simulink model "template_KR4_PreRTHS"  (Simulink 8.2)
settings: Solver=FixedStepDiscrete  StartTime=0.0  StopTime=RunningTime  FixedStep=sample  RelTol=1e-3
undefined symbols (not defined in the file): ElementsStruct, Integrator, NumFreeDOF, RigidLinkMasterMatrix, RigidLinkNo, RigidLinkNodeID, RigidLinkSlaveMatrix, sample, SampleRate, Structure
libraries: HybridFEMLibrary x2
(part 1 of 2)
CloseFcn:
  | rtwprivate ssgencode ModelCloseRequest hybriddaq1dof
settings Model: MinMaxOverflowLogging=ForceOff  Creator=RTMD  LastModifiedBy=Thomas Marullo  BufferReuse=off
settings DataIOCC: LimitDataPoints=off
settings OptimizationCC: BlockReduction=off  OptimizeBlockIOStorage=off  BufferReuse=off  ExpressionFolding=off  LocalBlockOutputs=off  InitFltsAndDblsToZero=on
settings DebuggingCC: SignalResolutionControl=TryResolveAllWithWarning  MultiTaskDSMMsg=warning  FcnCallInpInsideContextMsg=EnableAllAsWarning
settings HardwareCC: ProdIntDivRoundTo=Zero  ProdEndianess=LittleEndian  ProdHWDeviceType=Generic->32-bit x86 compatible
settings SFSimCC: SimParseCustomCode=off
settings RTWCC: ProcessScript=grt_make_rtw_hook
settings GRTTargetCC: CombineOutputUpdateFcns=on  GRTInterface=off

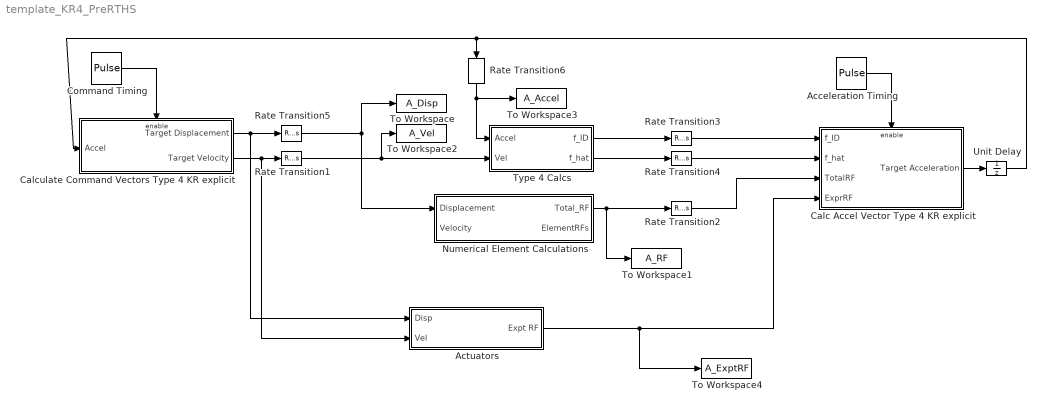
== system template_KR4_PreRTHS ==
  Acceleration Timing : DiscretePulseGenerator  Period=Integrator.Interpolations  PhaseDelay=Integrator.Interpolations-1  SampleTime=sample
  Actuators : Subsystem
  Calc Accel Vector Type 4 KR explicit : Subsystem
  Calculate Command Vectors Type 4 KR explicit : Subsystem  TreatAsAtomicUnit=on  SystemSampleTime=SampleRate
  Command Timing : DiscretePulseGenerator  Period=Integrator.Interpolations  SampleTime=sample
  Numerical Element Calculations : MATLAB Function  TreatAsAtomicUnit=on
  Rate Transition1 : RateTransition  Deterministic=off  OutPortSampleTime=SampleRate
  Rate Transition2 : RateTransition  Deterministic=off  OutPortSampleTime=sample
  Rate Transition3 : RateTransition  Deterministic=off  OutPortSampleTime=sample
  Rate Transition4 : RateTransition  Deterministic=off  OutPortSampleTime=sample
  Rate Transition5 : RateTransition  Deterministic=off  OutPortSampleTime=SampleRate
  Rate Transition6 : RateTransition  Deterministic=off  OutPortSampleTime=SampleRate
  To Workspace : ToWorkspace  VariableName=A_Disp  SampleTime=-1
  To Workspace1 : ToWorkspace  VariableName=A_RF  SampleTime=-1
  To Workspace2 : ToWorkspace  VariableName=A_Vel  SampleTime=-1
  To Workspace3 : ToWorkspace  VariableName=A_Accel  SampleTime=-1
  To Workspace4 : ToWorkspace  VariableName=A_ExptRF  SampleTime=-1
  Type 4 Calcs : Subsystem  TreatAsAtomicUnit=on  SystemSampleTime=SampleRate
  Unit Delay : UnitDelay  InitialCondition=Integrator.Acceleration  SampleTime=-1
  wires:
  Acceleration Timing/1 -> Calc Accel Vector Type 4 KR explicit/Enable
  Calculate Command Vectors Type 4 KR explicit/2(Target Velocity) -> Rate Transition1/1, Actuators/2(Vel)
  Rate Transition2/1 -> Calc Accel Vector Type 4 KR explicit/3(TotalRF)
  Command Timing/1 -> Calculate Command Vectors Type 4 KR explicit/Enable
  Calculate Command Vectors Type 4 KR explicit/1(Target Displacement) -> Rate Transition5/1, Actuators/1(Disp)
  Rate Transition5/1 -> Numerical Element Calculations/1(Displacement), To Workspace/1
  Unit Delay/1 -> Rate Transition6/1, Calculate Command Vectors Type 4 KR explicit/1(Accel)
  Rate Transition3/1 -> Calc Accel Vector Type 4 KR explicit/1(f_ID)
  Numerical Element Calculations/1(Total_RF) -> Rate Transition2/1, To Workspace1/1
  Rate Transition1/1 -> Type 4 Calcs/2(Vel), To Workspace2/1
  Calc Accel Vector Type 4 KR explicit/1(Target Acceleration) -> Unit Delay/1
  Type 4 Calcs/1(f_ID) -> Rate Transition3/1
  Type 4 Calcs/2(f_hat) -> Rate Transition4/1
  Rate Transition6/1 -> Type 4 Calcs/1(Accel), To Workspace3/1
  Rate Transition4/1 -> Calc Accel Vector Type 4 KR explicit/2(f_hat)
  Actuators/1(Expt RF) -> To Workspace4/1, Calc Accel Vector Type 4 KR explicit/4(ExprRF)

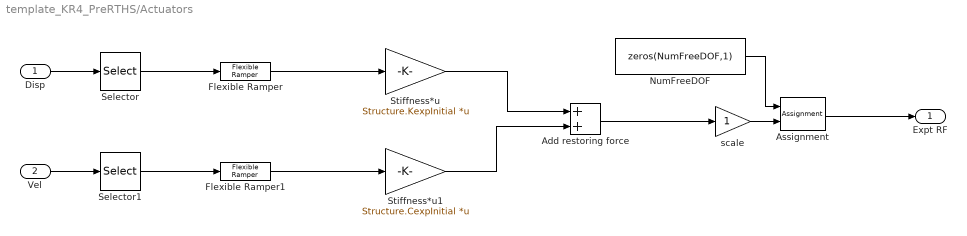
== system template_KR4_PreRTHS/Actuators ==
  Disp : Inport
  Vel : Inport  Port=2
  Add restoring force : Sum
  Assignment : Assignment  IndexOptions=Index vector (dialog)  Indices=Structure.InterfaceDOF  OutputSizes=1
  Flexible Ramper : HybridFEMLibrary/Flexible Ramper  ramps=Integrator.Interpolations  samplerate=sample  initVal=zeros(size(Structure.InterfaceDOF),1)
  Flexible Ramper1 : HybridFEMLibrary/Flexible Ramper  ramps=Integrator.Interpolations  samplerate=sample  initVal=zeros(size(Structure.InterfaceDOF),1)
  NumFreeDOF : Constant  Value=zeros(NumFreeDOF,1)
  Selector : Selector  InputPortWidth=NumFreeDOF  IndexOptions=Index vector (dialog)  Indices=Structure.InterfaceDOF  OutputSizes=1
  Selector1 : Selector  InputPortWidth=NumFreeDOF  IndexOptions=Index vector (dialog)  Indices=Structure.InterfaceDOF  OutputSizes=1
  Stiffness*u : Gain  Gain=Structure.KexpInitial  Multiplication=Matrix(K*u) (u vector)
  Stiffness*u1 : Gain  Gain=Structure.CexpInitial  Multiplication=Matrix(K*u) (u vector)
  scale : Gain
  Expt RF : Outport
  wires:
  Flexible Ramper1/1 -> Stiffness*u1/1
  Flexible Ramper/1 -> Stiffness*u/1
  Stiffness*u1/1 -> Add restoring force/2
  scale/1 -> Assignment/2
  NumFreeDOF/1 -> Assignment/1
  Add restoring force/1 -> scale/1
  Stiffness*u/1 -> Add restoring force/1
  Assignment/1 -> Expt RF/1
  Selector1/1 -> Flexible Ramper1/1
  Selector/1 -> Flexible Ramper/1
  Vel/1 -> Selector1/1
  Disp/1 -> Selector/1

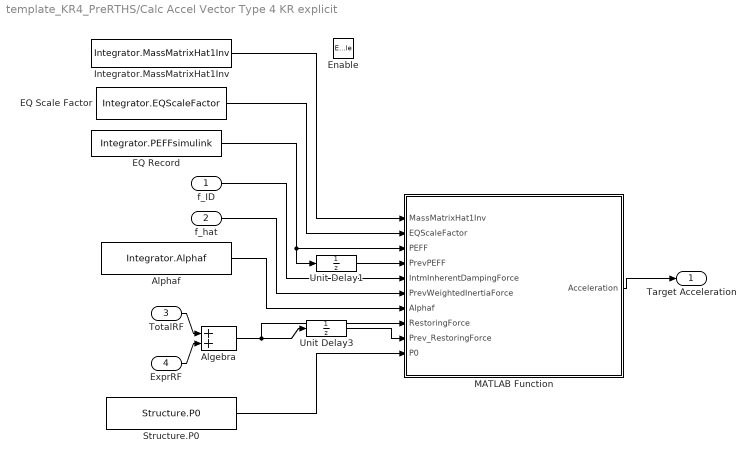
== system template_KR4_PreRTHS/Calc Accel Vector Type 4 KR explicit ==
  f_ID : Inport
  f_hat : Inport  Port=2
  TotalRF : Inport  Port=3
  ExprRF : Inport  Port=4
  Enable : EnablePort
  Algebra : Sum
  Alphaf : Constant  Value=Integrator.Alphaf
  EQ Record : FromWorkspace  VariableName=Integrator.PEFFsimulink  Interpolate=off  OutputAfterFinalValue=Holding final value
  EQ Scale Factor : Constant  Value=Integrator.EQScaleFactor
  Integrator.MassMatrixHat1Inv : Constant  Value=Integrator.MassMatrixHat1Inv
  MATLAB Function : MATLAB Function  TreatAsAtomicUnit=on
  Structure.P0 : Constant  Value=Structure.P0
  Unit Delay1 : UnitDelay  InitialCondition=Integrator.PEFF(1,:)  SampleTime=-1
  Unit Delay3 : UnitDelay  InitialCondition=Integrator.RestoringForce  SampleTime=-1
  Target Acceleration : Outport
  wires:
  Unit Delay1/1 -> MATLAB Function/4(PrevPEFF)
  TotalRF/1 -> Algebra/1
  ExprRF/1 -> Algebra/2
  Integrator.MassMatrixHat1Inv/1 -> MATLAB Function/1(MassMatrixHat1Inv)
  EQ Record/1 -> Unit Delay1/1, MATLAB Function/3(PEFF)
  f_ID/1 -> MATLAB Function/5(IntmInherentDampingForce)
  f_hat/1 -> MATLAB Function/6(PrevWeightedInertiaForce)
  Alphaf/1 -> MATLAB Function/7(Alphaf)
  Algebra/1 -> MATLAB Function/8(RestoringForce), Unit Delay3/1
  Unit Delay3/1 -> MATLAB Function/9(Prev_RestoringForce)
  Structure.P0/1 -> MATLAB Function/10(P0)
  MATLAB Function/1(Acceleration) -> Target Acceleration/1
  EQ Scale Factor/1 -> MATLAB Function/2(EQScaleFactor)

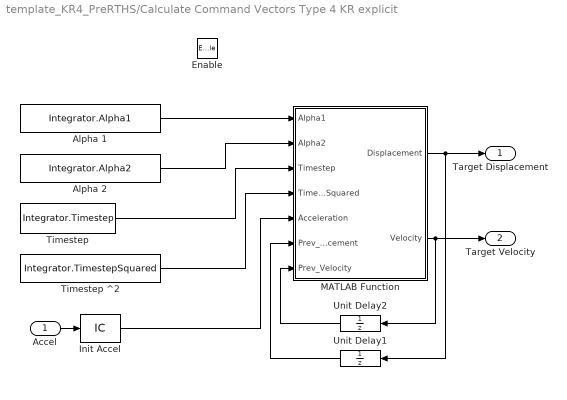
== system template_KR4_PreRTHS/Calculate Command Vectors Type 4 KR explicit ==
  Accel : Inport
  Enable : EnablePort
  Alpha 1 : Constant  Priority=5  Value=Integrator.Alpha1
  Alpha 2 : Constant  Priority=11  Value=Integrator.Alpha2
  Init Accel : InitialCondition  Priority=2  Value=Integrator.Acceleration
  MATLAB Function : MATLAB Function  TreatAsAtomicUnit=on
  "Timestep " : Constant  Priority=3  Value=Integrator.Timestep
  Timestep ^2 : Constant  Priority=9  Value=Integrator.TimestepSquared
  Unit Delay1 : UnitDelay  Priority=7  InitialCondition=Integrator.Displacement  SampleTime=-1
  Unit Delay2 : UnitDelay  Priority=7  InitialCondition=Integrator.Velocity  SampleTime=-1
  Target Displacement : Outport
  Target Velocity : Outport  Port=2
  wires:
  Accel/1 -> Init Accel/1
  MATLAB Function/1(Displacement) -> Target Displacement/1, Unit Delay1/1
  MATLAB Function/2(Velocity) -> Target Velocity/1, Unit Delay2/1
  Unit Delay1/1 -> MATLAB Function/6(Prev_Displacement)
  Unit Delay2/1 -> MATLAB Function/7(Prev_Velocity)
  Alpha 1/1 -> MATLAB Function/1(Alpha1)
  Alpha 2/1 -> MATLAB Function/2(Alpha2)
  "Timestep "/1 -> MATLAB Function/3(Timestep)
  Timestep ^2/1 -> MATLAB Function/4(TimestepSquared)
  Init Accel/1 -> MATLAB Function/5(Acceleration)

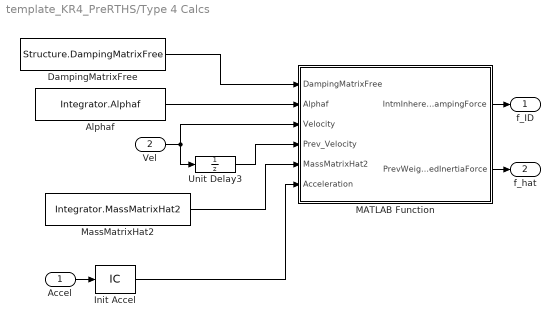
== system template_KR4_PreRTHS/Type 4 Calcs ==
  Accel : Inport
  Vel : Inport  Port=2
  Alphaf : Constant  Value=Integrator.Alphaf
  DampingMatrixFree : Constant  Value=Structure.DampingMatrixFree
  Init Accel : InitialCondition  Value=Integrator.Acceleration
  MATLAB Function : MATLAB Function  TreatAsAtomicUnit=on
  MassMatrixHat2 : Constant  Value=Integrator.MassMatrixHat2
  Unit Delay3 : UnitDelay  InitialCondition=Integrator.Velocity  SampleTime=-1
  f_ID : Outport
  f_hat : Outport  Port=2
  wires:
  Vel/1 -> Unit Delay3/1, MATLAB Function/3(Velocity)
  Accel/1 -> Init Accel/1
  MATLAB Function/1(IntmInherentDampingForce) -> f_ID/1
  MATLAB Function/2(PrevWeightedInertiaForce) -> f_hat/1
  DampingMatrixFree/1 -> MATLAB Function/1(DampingMatrixFree)
  Alphaf/1 -> MATLAB Function/2(Alphaf)
  Unit Delay3/1 -> MATLAB Function/4(Prev_Velocity)
  MassMatrixHat2/1 -> MATLAB Function/5(MassMatrixHat2)
  Init Accel/1 -> MATLAB Function/6(Acceleration)
